simulink model "za muameera"  (R2017b)
settings: Solver=VariableStepAuto  StartTime=0.0  StopTime=800  RelTol=1e-3
undefined symbols (not defined in the file): ln
libraries: simulink x14
settings Model: Creator=DT User  LastModifiedBy=DT User

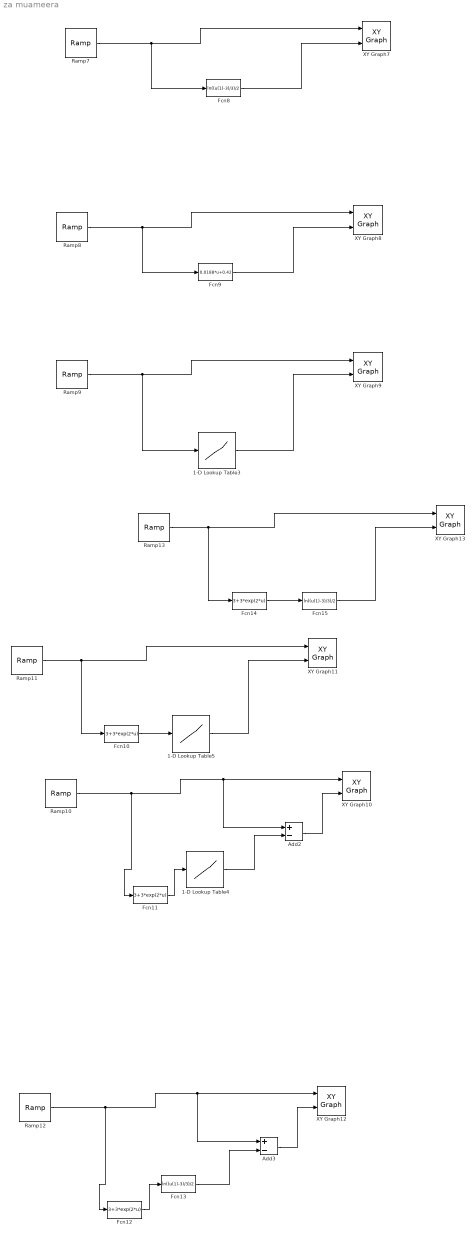
== system za muameera ==
  1-D Lookup Table3 : Lookup_n-D  NumberOfTableDimensions=1  BreakpointsForDimension1=3+3*exp(2*[0:5:50])  Table=[0:5:50]  InternalRulePriority=Speed  RndMeth=Simplest  InputSameDT=on
  1-D Lookup Table4 : Lookup_n-D  NumberOfTableDimensions=1  BreakpointsForDimension1=3+3*exp(2*[0:5:50])  Table=[0:5:50]  InternalRulePriority=Speed  RndMeth=Simplest  InputSameDT=on
  1-D Lookup Table5 : Lookup_n-D  NumberOfTableDimensions=1  BreakpointsForDimension1=3+3*exp(2*[0:5:50])  Table=[0:5:50]  InternalRulePriority=Speed  RndMeth=Simplest  InputSameDT=on
  Add2 : Sum  Inputs=+-
  Add3 : Sum  Inputs=+-
  Fcn{10..12,14} (4 alike) : Fcn  Expr=3+3*exp(2*u)
  Fcn13 : Fcn  Expr=ln((u(1)-3)/3)/2
  Fcn15 : Fcn  Expr=ln((u(1)-3)/3)/2
  Fcn8 : Fcn  Expr=ln((u(1)-3)/3)/2
  Fcn9 : Fcn  Expr=0.0188*u+0.42
  Ramp{7..13} (7 alike) : simulink/Sources/Ramp  slope=1  start=0  X0=0
  XY Graph10 : simulink/Sinks/XY Graph  xmin=0  xmax=50  ymin=-10  ymax=10  st=1
  XY Graph11 : simulink/Sinks/XY Graph  xmin=0  xmax=50  ymin=-10  ymax=100  st=1
  XY Graph12 : simulink/Sinks/XY Graph  xmin=0  xmax=50  ymin=-10  ymax=10  st=1
  XY Graph13 : simulink/Sinks/XY Graph  xmin=0  xmax=50  ymin=-10  ymax=100  st=1
  XY Graph7 : simulink/Sinks/XY Graph  xmin=0  xmax=50  ymin=0  ymax=2  st=1
  XY Graph8 : simulink/Sinks/XY Graph  xmin=0  xmax=50  ymin=0  ymax=2  st=1
  XY Graph9 : simulink/Sinks/XY Graph  xmin=0  xmax=50  ymin=-10  ymax=10  st=1
  wires:
  Fcn8/1 -> XY Graph7/2
  1-D Lookup Table3/1 -> XY Graph9/2
  Add3/1 -> XY Graph12/2
  Ramp12/1 -> XY Graph12/1, Add3/1, Fcn12/1
  Ramp11/1 -> Fcn10/1, XY Graph11/1
  Add2/1 -> XY Graph10/2
  1-D Lookup Table4/1 -> Add2/2
  Ramp7/1 -> Fcn8/1, XY Graph7/1
  Fcn11/1 -> 1-D Lookup Table4/1
  1-D Lookup Table5/1 -> XY Graph11/2
  Fcn9/1 -> XY Graph8/2
  Ramp8/1 -> XY Graph8/1, Fcn9/1
  Ramp9/1 -> 1-D Lookup Table3/1, XY Graph9/1
  Fcn13/1 -> Add3/2
  Ramp13/1 -> XY Graph13/1, Fcn14/1
  Fcn12/1 -> Fcn13/1
  Fcn15/1 -> XY Graph13/2
  Fcn10/1 -> 1-D Lookup Table5/1
  Ramp10/1 -> Fcn11/1, Add2/1, XY Graph10/1
  Fcn14/1 -> Fcn15/1
